simulink model "Binary_ASK_Modulation"  (R2024a)
settings: Solver=VariableStepAuto  StartTime=0.0  StopTime=10.0  RelTol=1e-3
libraries: commrandsrc3 x1, commfilt2 x1
settings Model: Creator=alice  LastModifiedBy=alice

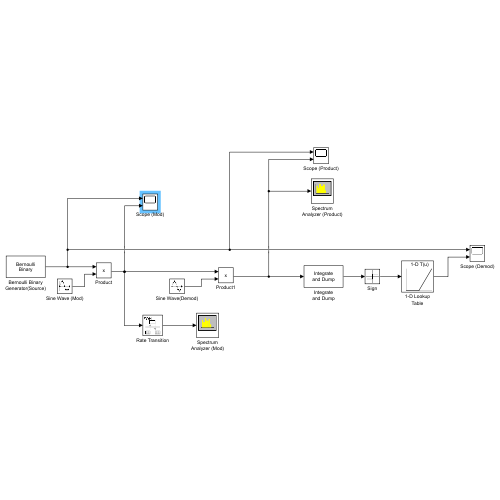
[thumbnail: Simulink's stored preview of the top-level diagram]
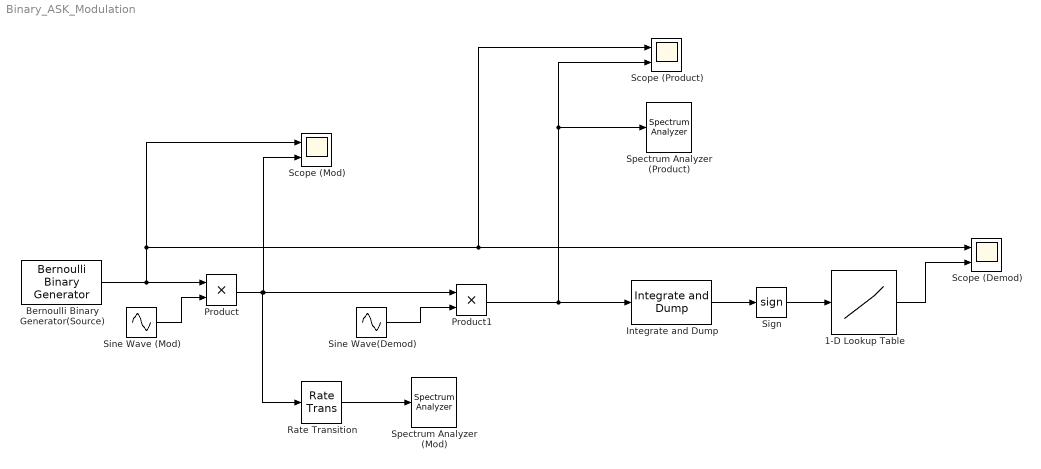
== system Binary_ASK_Modulation ==
  1-D Lookup Table : Lookup_n-D  NumberOfTableDimensions=1  BreakpointsForDimension1=[-1,0,1]  Table=[0,0,1]  InternalRulePriority=Speed  RndMeth=Simplest
  Bernoulli Binary Generator(Source) : commrandsrc3/Bernoulli Binary Generator  ProbabilityOfZero=0.5  SeedSource=Parameter  Seed=67  SampleTime=1e-3  SamplesPerFrame=1  OutputDataType=double  SimulateUsing=Interpreted execution
  Integrate and Dump : commfilt2/Integrate and Dump  obssamples=8  offsetsamples=0  nodump=off  roundingMode=Floor  overflowMode=off  outputDataTypeStr=Inherit: Same as accumulator  outputLastDataTypeStr=Inherit: Same as accumulator
  Product : Product
  Product1 : Product
  Rate Transition : RateTransition  OutPortSampleTime=0.5e-4
  Scope (Demod) : Scope  NumInputPorts=2
  Scope (Mod) : Scope  NumInputPorts=2
  Scope (Product) : Scope  NumInputPorts=2
  Sign : Signum
  Sine Wave (Mod) : Sin  SineType=Sample based  Samples=5000  SampleTime=1e-7
  Sine Wave(Demod) : Sin  SineType=Sample based  Samples=5000  SampleTime=1e-7
  Spectrum Analyzer (Mod) : SpectrumAnalyzer  WindowPosition=[1.000000,49.000000,1280.000000,729.000000,]  ScopeFrameLocation=window  YLimits=[-81.05442386995875,49.946620992749295]  SelectedToolstripTab=spectrumAnalyzerToolstrip.channelMeasurementsTab
  Spectrum Analyzer (Product) : SpectrumAnalyzer  WindowPosition=[240.000000,150.000000,800.000000,500.000000,]  ScopeFrameLocation=window  YLimits=[-253.22098246,55.74557046]
  wires:
  Bernoulli Binary Generator(Source)/1 -> Scope (Product)/1, Scope (Demod)/1, Scope (Mod)/1, Product/1
  Sine Wave (Mod)/1 -> Product/2
  Product/1 -> Product1/1, Scope (Mod)/2, Rate Transition/1
  Rate Transition/1 -> Spectrum Analyzer (Mod)/1
  Sine Wave(Demod)/1 -> Product1/2
  Product1/1 -> Integrate and Dump/1, Spectrum Analyzer (Product)/1, Scope (Product)/2
  Integrate and Dump/1 -> Sign/1
  Sign/1 -> 1-D Lookup Table/1
  1-D Lookup Table/1 -> Scope (Demod)/2
